simulink subsystem "Gyroscope"  (R2022a)
settings: Solver=VariableStepAuto  StartTime=0.0  StopTime=10.0  RelTol=1e-3
values from neighbouring files (symbols this model uses):
  ARW = sqrt(N_ARW^2)    [backend.m]
  RRW = sqrt(K_RRW^2/3)    [backend.m]
libraries: matrix_library x1
settings Model: Creator=emmamarsden  LastModifiedBy=emmamarsden

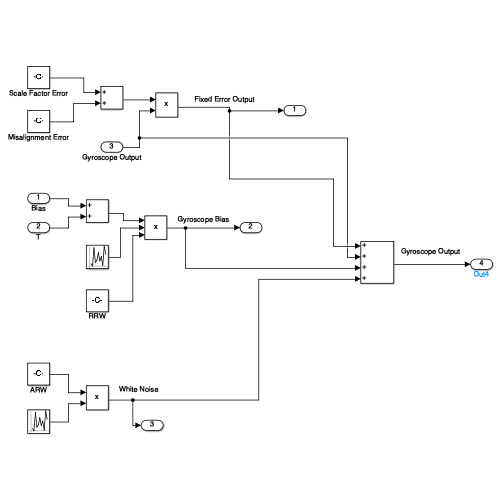
[thumbnail: Simulink's stored preview of the top-level diagram]
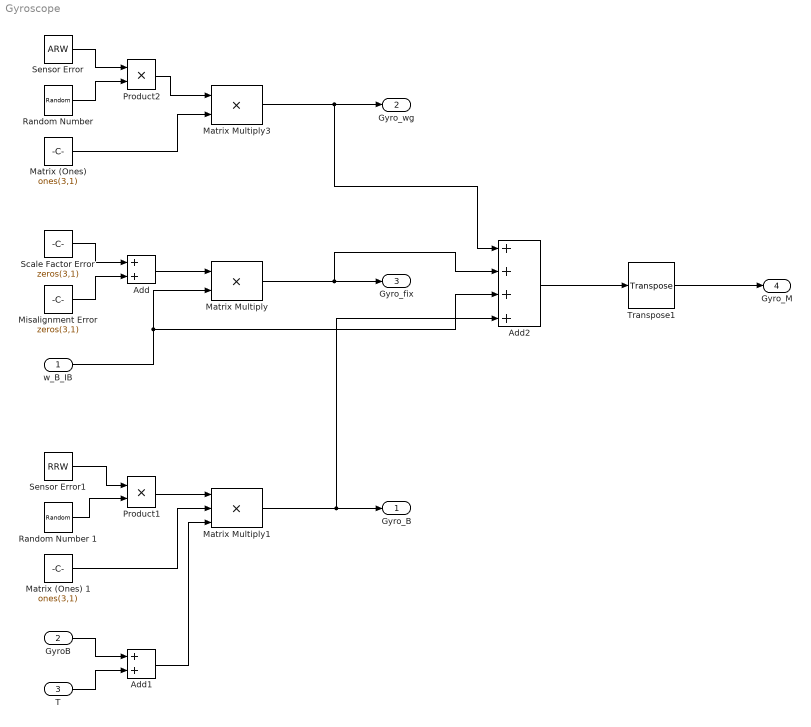
== system Gyroscope ==
  w_B_IB : Inport
  GyroB : Inport  Port=2
  T : Inport  Port=3
  Add : Sum
  Add1 : Sum
  Add2 : Sum  Inputs=++++
  Matrix (Ones) : Constant  Value=ones(3,1)  VectorParams1D=off
  Matrix (Ones) 1 : Constant  Value=ones(3,1)  VectorParams1D=off
  Matrix Multiply : Product
  Matrix Multiply1 : Product  Inputs=3
  Matrix Multiply3 : Product
  Misalignment Error : Constant  Value=zeros(3,1)
  Product1 : Product
  Product2 : Product
  Random Number : UniformRandomNumber  SampleTime=0.1
  Random Number 1 : UniformRandomNumber  SampleTime=0.1
  Scale Factor Error : Constant  Value=zeros(3,1)
  Sensor Error : Constant  Value=ARW
  Sensor Error1 : Constant  Value=RRW
  Transpose1 : matrix_library/Transpose
      settings: SourceProductBaseCode=SL
  Gyro_B : Outport
  Gyro_wg : Outport  Port=2
  Gyro_fix : Outport  Port=3
  Gyro_M : Outport  Port=4
  wires:
  Add/1 -> Matrix Multiply/1
  Scale Factor Error/1 -> Add/1
  Misalignment Error/1 -> Add/2
  Random Number/1 -> Product2/2
  Sensor Error/1 -> Product2/1
  Product2/1 -> Matrix Multiply3/1
  Matrix (Ones)/1 -> Matrix Multiply3/2
  Matrix Multiply3/1 -> Gyro_wg/1, Add2/1
  Random Number 1/1 -> Product1/2
  Sensor Error1/1 -> Product1/1
  Matrix (Ones) 1/1 -> Matrix Multiply1/2
  Product1/1 -> Matrix Multiply1/1
  Matrix Multiply/1 -> Gyro_fix/1, Add2/2
  T/1 -> Add1/2
  GyroB/1 -> Add1/1
  Add1/1 -> Matrix Multiply1/3
  Matrix Multiply1/1 -> Add2/4, Gyro_B/1
  w_B_IB/1 -> Matrix Multiply/2, Add2/3
  Add2/1 -> Transpose1/1
  Transpose1/1 -> Gyro_M/1
